simulink model "prblm5"  (R2020b)
settings: Solver=VariableStepAuto  StartTime=0.0  StopTime=10.0  RelTol=1e-3
model workspace (MAT data in the model file):
  C = Simulink.Parameter
  C.Value = 1e-05
  C.DataType = 'auto'
  C.Dimensions = [1 1]
  R = Simulink.Parameter
  R.Value = 10
  R.DataType = 'auto'
  R.Dimensions = [1 1]
settings Model: Creator=Dell  LastModifiedBy=Dell

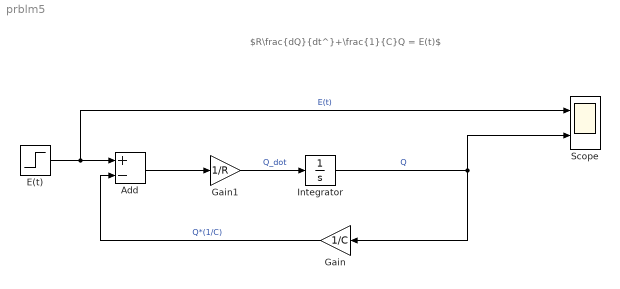
== system prblm5 ==
  note: $R\frac{dQ}{dt^}+\frac{1}{C}Q = E(t)$
  Add : Sum  Inputs=+-
  E(t) : Step  After=3  SampleTime=0
  Gain : Gain  Gain=1/C
  Gain1 : Gain  Gain=1/R
  Integrator : Integrator  InitialCondition=0.001
  Scope : Scope  NumInputPorts=2
  wires:
  Gain1/1 -> Integrator/1  "Q_dot"
  Integrator/1 -> Scope/2, Gain/1  "Q"
  Add/1 -> Gain1/1
  Gain/1 -> Add/2  "Q*(1/C)"
  E(t)/1 -> Scope/1, Add/1  "E(t)"
